simulink model "Blink_Led"  (R2024b)
settings: Solver=VariableStepAuto  StartTime=0.0  StopTime=10.0  RelTol=1e-3
settings Model: Creator=Ahmad  LastModifiedBy=Ahmad

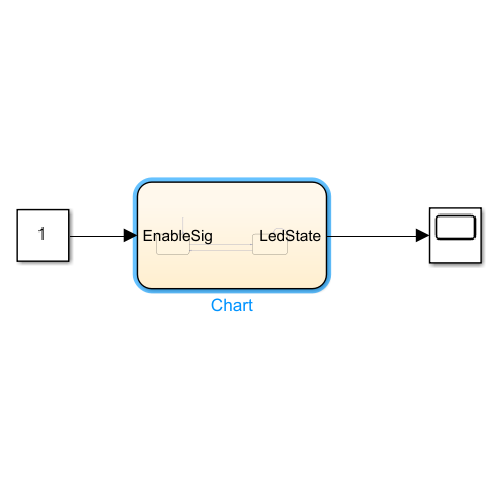
[thumbnail: Simulink's stored preview of the top-level diagram]
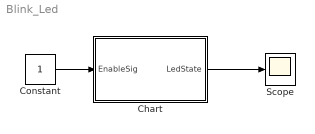
== system Blink_Led ==
  Chart : Stateflow chart  TreatAsAtomicUnit=on
  Constant : Constant
  Scope : Scope
  wires:
  Chart/1(LedState) -> Scope/1
  Constant/1 -> Chart/1(EnableSig)

== stateflow chart Blink_Led/Chart ==
  state LedOff
    entry:
    LedState=0;
  state LedOn
    entry:
    LedState=1;
  (default) -> LedOff
  LedOn -> LedOn [order 2] : [EnableSig==0]
  LedOff -> LedOn : after(1,sec)
  LedOn -> LedOff [order 1] : after(1,sec)[EnableSig==1]
  data: LedState output; EnableSig input
